simulink model "item1b"  (R2019a)
settings: Solver=VariableStepAuto  StartTime=0.0  StopTime=20  RelTol=1e-3
libraries: simulink x2
settings Model: Creator=Usuario  LastModifiedBy=Usuario

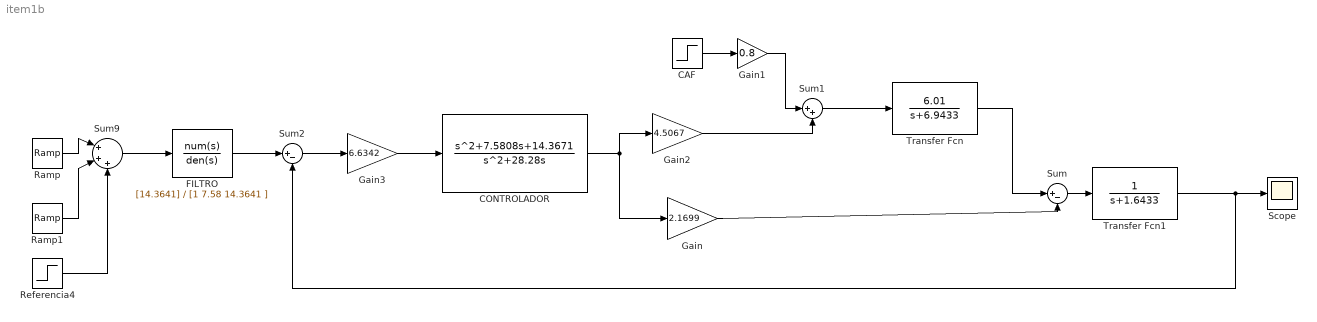
== system item1b ==
  CAF : Step  Time=10  Before=5.1  After=5.1  SampleTime=0.01
  "CONTROLADOR " : TransferFcn  Numerator=[1 7.5808 14.3671]  Denominator=[1 28.28 0]
  "FILTRO " : TransferFcn  Numerator=[14.3641]  Denominator=[1 7.58 14.3641 ]
  Gain : Gain  Gain=2.1699
  Gain1 : Gain  Gain=0.8
  Gain2 : Gain  Gain=4.5067
  Gain3 : Gain  Gain=6.6342
  Ramp : simulink/Sources/Ramp  slope=2.345/5  start=0  InitialOutput=0
  Ramp1 : simulink/Sources/Ramp  slope=-2.345/5  start=5  InitialOutput=0
  Referencia4 : Step  Time=10  After=0.1  SampleTime=0.01
  Scope : Scope
  Sum : Sum  Inputs=|+-
  Sum1 : Sum  Inputs=|++
  Sum2 : Sum  Inputs=|+-
  Sum9 : Sum  Inputs=|+++
  Transfer Fcn : TransferFcn  Numerator=[6.01]  Denominator=[1 6.9433]
  Transfer Fcn1 : TransferFcn  Denominator=[1 1.6433]
  wires:
  Sum/1 -> Transfer Fcn1/1
  Transfer Fcn/1 -> Sum/1
  Gain1/1 -> Sum1/1
  Gain2/1 -> Sum1/2
  Sum1/1 -> Transfer Fcn/1
  Gain/1 -> Sum/2
  Gain3/1 -> "CONTROLADOR "/1
  "CONTROLADOR "/1 -> Gain/1, Gain2/1
  CAF/1 -> Gain1/1
  Sum2/1 -> Gain3/1
  Transfer Fcn1/1 -> Sum2/2, Scope/1
  Ramp/1 -> Sum9/1
  Ramp1/1 -> Sum9/2
  Referencia4/1 -> Sum9/3
  Sum9/1 -> "FILTRO "/1
  "FILTRO "/1 -> Sum2/1
